simulink subsystem "BEV4EM"  (R2023a)
settings: Solver=VariableStepAuto  StartTime=0.0  StopTime=10.0  RelTol=1e-3
undefined symbols (not defined in the file): PlntDriveshftDamp, PlntDriveshftStiff, PlntEM1RotDamp, PlntEM1RotInertia, PlntEM2RotDamp, PlntEM2RotInertia, PlntEM3RotDamp, PlntEM3RotInertia, PlntEM4RotDamp, PlntEM4RotInertia
libraries: autolibsharedcoupling x8
settings Model: Creator=The MathWorks, Inc.  LastModifiedBy=The MathWorks, Inc.
settings OptimizationCC: ReuseModelBlockBuffer=off
settings DebuggingCC: SubsystemReferenceDiagnosticForUnitTest=warning

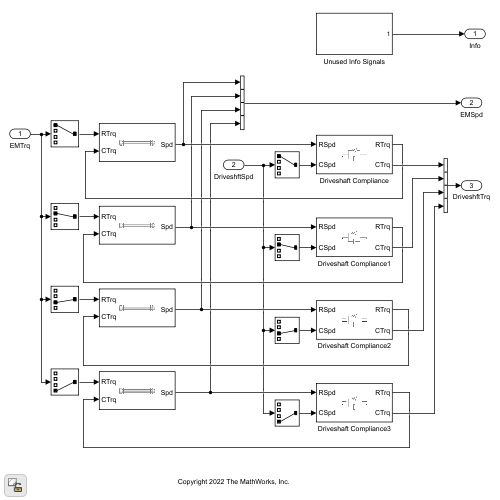
[thumbnail: Simulink's stored preview of the top-level diagram]
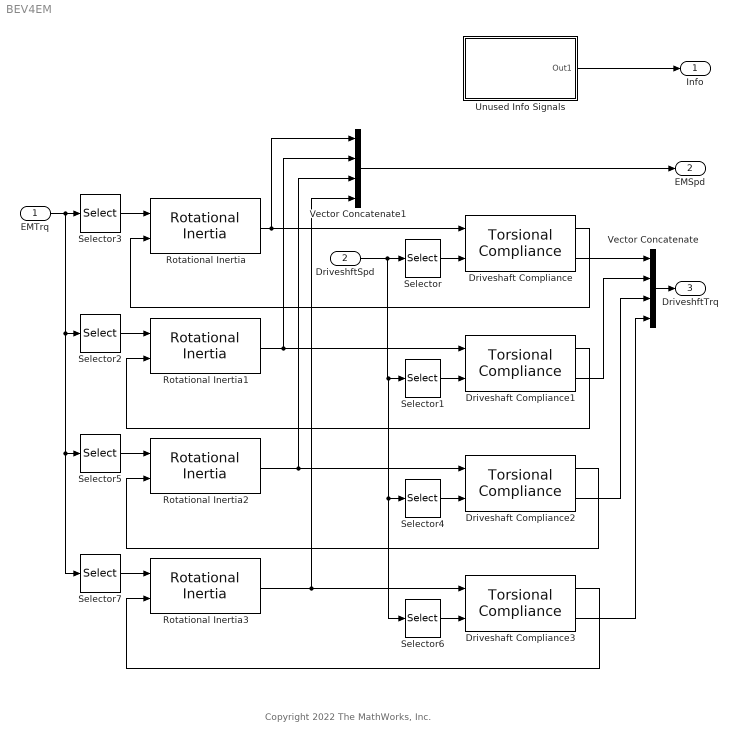
== system BEV4EM ==
  note: Copyright 2022 The MathWorks, Inc.
  EMTrq : Inport
  DriveshftSpd : Inport  Port=2
  Driveshaft Compliance{,1..3} (4 alike) : autolibsharedcoupling/Torsional Compliance  port_config=Simulink  extInfo=off  k=PlntDriveshftStiff  b=PlntDriveshftDamp  theta_o=PlntDriveshftInitDeflect  domega_o=PlntDriveshftInitVel  omega_c=PlntDriveshftDampCutoffFreq  blkID=0  aMode=1
  Rotational Inertia : autolibsharedcoupling/Rotational Inertia  port_config=Simulink  extInfo=off  externJ=off  J=PlntEM1RotInertia  b=PlntEM1RotDamp  omega_o=PlntEM1RotInitSpd  blkID=0  aMode=1
      settings: LibrarySourceBlock=autolibcoupling/Rotational Inertia
  Rotational Inertia1 : autolibsharedcoupling/Rotational Inertia  port_config=Simulink  extInfo=off  externJ=off  J=PlntEM2RotInertia  b=PlntEM2RotDamp  omega_o=PlntEM2RotInitSpd  blkID=0  aMode=1
      settings: LibrarySourceBlock=autolibcoupling/Rotational Inertia
  Rotational Inertia2 : autolibsharedcoupling/Rotational Inertia  port_config=Simulink  extInfo=off  externJ=off  J=PlntEM3RotInertia  b=PlntEM3RotDamp  omega_o=PlntEM3RotInitSpd  blkID=0  aMode=1
      settings: LibrarySourceBlock=autolibcoupling/Rotational Inertia
  Rotational Inertia3 : autolibsharedcoupling/Rotational Inertia  port_config=Simulink  extInfo=off  externJ=off  J=PlntEM4RotInertia  b=PlntEM4RotDamp  omega_o=PlntEM4RotInitSpd  blkID=0  aMode=1
      settings: LibrarySourceBlock=autolibcoupling/Rotational Inertia
  Selector : Selector  InputPortWidth=4  IndexOptions=Index vector (dialog)  Indices=[1]  OutputSizes=1
  Selector1 : Selector  InputPortWidth=4  IndexOptions=Index vector (dialog)  Indices=[2]  OutputSizes=1
  Selector2 : Selector  InputPortWidth=4  IndexOptions=Index vector (dialog)  Indices=[2]  OutputSizes=1
  Selector3 : Selector  InputPortWidth=4  IndexOptions=Index vector (dialog)  Indices=[1]  OutputSizes=1
  Selector4 : Selector  InputPortWidth=4  IndexOptions=Index vector (dialog)  Indices=[3]  OutputSizes=1
  Selector5 : Selector  InputPortWidth=4  IndexOptions=Index vector (dialog)  Indices=[3]  OutputSizes=1
  Selector6 : Selector  InputPortWidth=4  IndexOptions=Index vector (dialog)  Indices=[4]  OutputSizes=1
  Selector7 : Selector  InputPortWidth=4  IndexOptions=Index vector (dialog)  Indices=[4]  OutputSizes=1
  Unused Info Signals : Subsystem
  Vector Concatenate : Concatenate  NumInputs=4
  Vector Concatenate1 : Concatenate  NumInputs=4
  Info : Outport  VectorParamsAs1DForOutWhenUnconnected=off  BusOutputAsStruct=on
  EMSpd : Outport  Port=2  VectorParamsAs1DForOutWhenUnconnected=off  BusOutputAsStruct=on
  DriveshftTrq : Outport  Port=3  VectorParamsAs1DForOutWhenUnconnected=off
  wires:
  Vector Concatenate1/1 -> EMSpd/1
  Selector2/1 -> Rotational Inertia1/1
  Selector3/1 -> Rotational Inertia/1
  Vector Concatenate/1 -> DriveshftTrq/1
  Driveshaft Compliance1/2 -> Vector Concatenate/2
  Selector/1 -> Driveshaft Compliance/2
  Rotational Inertia1/1 -> Driveshaft Compliance1/1, Vector Concatenate1/2
  Driveshaft Compliance/2 -> Vector Concatenate/1
  Driveshaft Compliance/1 -> Rotational Inertia/2
  Driveshaft Compliance1/1 -> Rotational Inertia1/2
  Rotational Inertia/1 -> Driveshaft Compliance/1, Vector Concatenate1/1
  Selector1/1 -> Driveshaft Compliance1/2
  Unused Info Signals/1(Out1) -> Info/1
  Selector4/1 -> Driveshaft Compliance2/2
  Driveshaft Compliance2/1 -> Rotational Inertia2/2
  Rotational Inertia2/1 -> Driveshaft Compliance2/1, Vector Concatenate1/3
  Driveshaft Compliance2/2 -> Vector Concatenate/3
  Selector5/1 -> Rotational Inertia2/1
  Selector7/1 -> Rotational Inertia3/1
  Driveshaft Compliance3/2 -> Vector Concatenate/4
  Rotational Inertia3/1 -> Driveshaft Compliance3/1, Vector Concatenate1/4
  DriveshftSpd/1 -> Selector6/1, Selector4/1, Selector1/1, Selector/1
  Driveshaft Compliance3/1 -> Rotational Inertia3/2
  Selector6/1 -> Driveshaft Compliance3/2
  EMTrq/1 -> Selector7/1, Selector5/1, Selector2/1, Selector3/1

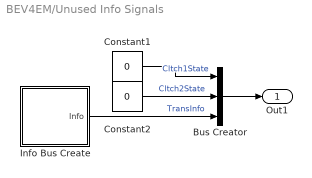
== system BEV4EM/Unused Info Signals ==
  Bus Creator : BusCreator  Inputs=3
  Constant1 : Constant  Value=0  SampleTime=-1
  Constant2 : Constant  Value=0  SampleTime=-1
  Info Bus Create : Subsystem
  Out1 : Outport
  wires:
  Constant2/1 -> Bus Creator/2  "Cltch2State"
  Constant1/1 -> Bus Creator/1  "Cltch1State"
  Bus Creator/1 -> Out1/1
  Info Bus Create/1(Info) -> Bus Creator/3  "TransInfo"

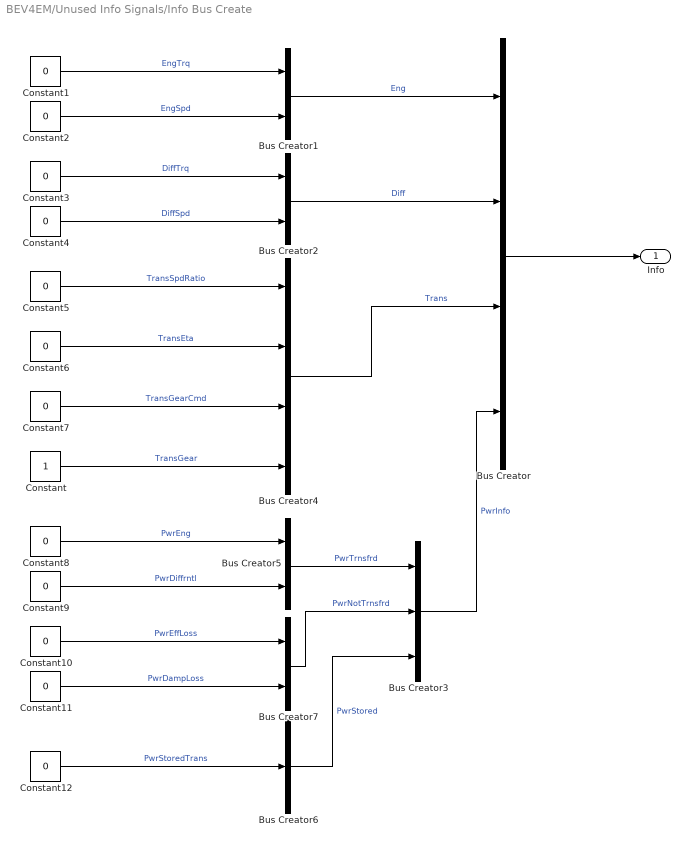
== system BEV4EM/Unused Info Signals/Info Bus Create ==
  Bus Creator : BusCreator  Inputs=4
  Bus Creator{1..2,5,7} (4 alike) : BusCreator  Inputs=2
  Bus Creator3 : BusCreator  Inputs=3
  Bus Creator4 : BusCreator  Inputs=4
  Bus Creator6 : BusCreator  Inputs=1
  Constant : Constant  SampleTime=-1
  Constant{1..12} (12 alike) : Constant  Value=0  SampleTime=-1
  Info : Outport
  wires:
  Bus Creator5/1 -> Bus Creator3/1  "PwrTrnsfrd"
  Bus Creator6/1 -> Bus Creator3/3  "PwrStored"
  Bus Creator7/1 -> Bus Creator3/2  "PwrNotTrnsfrd"
  Constant12/1 -> Bus Creator6/1  "PwrStoredTrans"
  Bus Creator2/1 -> Bus Creator/2  "Diff"
  Constant9/1 -> Bus Creator5/2  "PwrDiffrntl"
  Constant7/1 -> Bus Creator4/3  "TransGearCmd"
  Constant10/1 -> Bus Creator7/1  "PwrEffLoss"
  Constant1/1 -> Bus Creator1/1  "EngTrq"
  Constant5/1 -> Bus Creator4/1  "TransSpdRatio"
  Bus Creator/1 -> Info/1
  Constant3/1 -> Bus Creator2/1  "DiffTrq"
  Constant11/1 -> Bus Creator7/2  "PwrDampLoss"
  Constant/1 -> Bus Creator4/4  "TransGear"
  Constant2/1 -> Bus Creator1/2  "EngSpd"
  Bus Creator1/1 -> Bus Creator/1  "Eng"
  Constant6/1 -> Bus Creator4/2  "TransEta"
  Constant4/1 -> Bus Creator2/2  "DiffSpd"
  Constant8/1 -> Bus Creator5/1  "PwrEng"
  Bus Creator3/1 -> Bus Creator/4  "PwrInfo"
  Bus Creator4/1 -> Bus Creator/3  "Trans"
